simulink model "sampleModel62"  (R2021b)
settings: Solver=VariableStepAuto  StartTime=0.0  StopTime=10.0  RelTol=1e-3
undefined symbols (not defined in the file or in its folder): DiscIntNeverNeededParam, Newton, Raphson
libraries: simulink x13, slpidlib x3
settings Model: Creator=user  LastModifiedBy=user

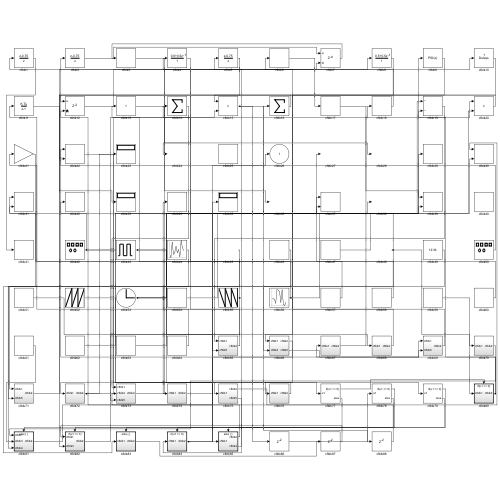
[thumbnail: Simulink's stored preview of the top-level diagram]
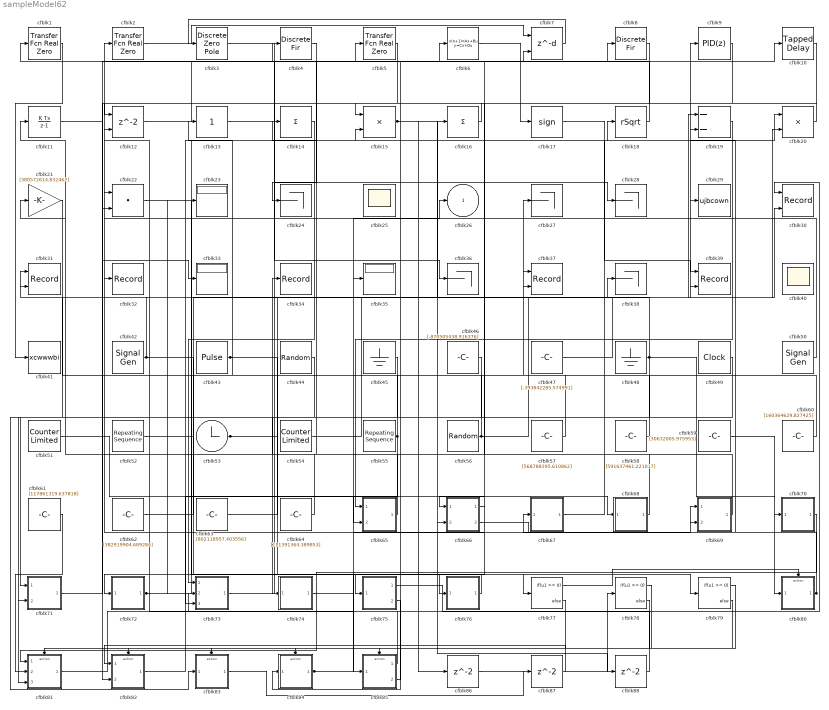
== system sampleModel62 ==
  cfblk1 : simulink/Discrete/Transfer Fcn Real Zero  ZeroZ=0.75  ICPrevInput=0.0  DoSatur=off
      settings: SourceProductBaseCode=SL
  cfblk10 : simulink/Discrete/Tapped Delay  vinit=0.0  samptime=-1  NumDelays=1  DelayOrder=Oldest  includeCurrent=off
  cfblk11 : DiscreteIntegrator  ICPrevOutput=DiscIntNeverNeededParam  ICPrevScaledInput=DiscIntNeverNeededParam
  cfblk12 : Delay  ShowEnablePort=on  SampleTime=1
      settings: InputPortMap=u0,e6
  cfblk13 : simulink/Math Operations/Slider Gain  gain=1  low=0  high=2
  cfblk14 : Sum  Inputs=+
  cfblk15 : Product  Inputs=**
  cfblk16 : Sum  Inputs=+
  cfblk17 : Signum
  cfblk18 : Sqrt  Operator=rSqrt  AlgorithmType=Newton-Raphson  SaturateOnIntegerOverflow=on
  cfblk19 : Sum  Inputs=--
  cfblk2 : simulink/Discrete/Transfer Fcn Real Zero  ZeroZ=0.75  ICPrevInput=0.0  DoSatur=off
      settings: SourceProductBaseCode=SL
  cfblk20 : Product
  cfblk21 : Gain  Gain=[380572614.832462]
  cfblk22 : DotProduct  InputSameDT=on  OutDataTypeStr=Inherit: Inherit via internal rule
  cfblk23 : Display
  cfblk{24,27..28,36,38} (5 alike) : Terminator
  cfblk25 : Scope
      settings: Floating=on
  cfblk29 : ToWorkspace  VariableName=ujbcown  SaveFormat=Timeseries  SampleTime=-1
  cfblk3 : DiscreteZeroPole  Poles=[0 0.5]  Gain=1
  cfblk30 : Record  FileSettingsInternal="{\"entries\":[{\"content\":{\"excelSettings\":{\"content\":{},\"type\":\"Streamout.ExcelSettings\"}},\"type\":\"Streamout.FileSettingStorage\",\"uuid\":\"89eb56b7-994b-4e5f-b351-745c7f58222d\"}],\"packageUris\":[\"http://schema.mathworks.com/mf0/streamout_blocks/R2020a\"],\"version\":\"1.0\"}"  Layout=[1 1]  SignalsInternal="{\"entries\":[{\"content\":{\"signals\":[{\"content\":{\"blockPath\":[\"sampleModel62/cfblk30\"],\"channel\":[],\"dimensions\":[1],\"domain\":\"sampleModel62/cfblk30\",\"lineColor\":\"#a2142f\",\"plots\":[1],\"port\":1,\"sid\":[\"\"],\"signalID\":2350,\"signalName\":\"cfblk75:1\"},\"type\":\"RecordBlkView.Signal\",\"uuid\":\"f3c1887c-4a82-4427-9ec1-d434c2a35077\"},{\"content\":{\"blockPath\":[\"sampleModel62/cfblk30\"],\"channel\":[],\"dimensions\":[1],\"domain\":\"sampleModel62/cfblk30\",\"lineColor\":\"#139fff\",\"plots\":[1],\"port\":2,\"sid\":[\"\"],\"signalID\":2354,\"signalName\":\"cfblk63\"},\"type\":\"RecordBlkView.Signal\",\"uuid\":\"385a4724-a655-411b-bda6-826876e1cbda\"}]},\"type\":\"RecordBlkView.InputSignals\",\"uuid\":\"7558fc44-3582-4613-9d91-3a130f029995\"}],\"packageUris\":[\"http://schema.mathworks.com/mf0/streamout_blocks/R2020a\"],\"version\":\"1.0\"}"  VisualizationBindings="{\"xyplotplugin\":{\"info\":[{\"series\":[{\"bindingParametersList\":[{\"parameter\":\"X-Axis\",\"signalID\":2350,\"signalName\":\"cfblk75:1\"},{\"parameter\":\"Y-Axis\",\"signalID\":2354,\"signalName\":\"cfblk63\"}],\"seriesID\":61633}],\"subplotID\":1}]}}"  CompatibilityTag=XY
  cfblk31 : Record  FileSettingsInternal="{\"entries\":[{\"content\":{\"excelSettings\":{\"content\":{},\"type\":\"Streamout.ExcelSettings\"}},\"type\":\"Streamout.FileSettingStorage\",\"uuid\":\"f6cec285-720d-4525-9b6c-a4037b512930\"}],\"packageUris\":[\"http://schema.mathworks.com/mf0/streamout_blocks/R2020a\"],\"version\":\"1.0\"}"  Layout=[1 1]  SignalsInternal="{\"entries\":[{\"content\":{\"signals\":[{\"content\":{\"blockPath\":[\"sampleModel62/cfblk31\"],\"channel\":[],\"dimensions\":[1],\"domain\":\"sampleModel62/cfblk31\",\"lineColor\":\"#139fff\",\"plots\":[1],\"port\":2,\"sid\":[\"\"],\"signalID\":2358,\"signalName\":\"cfblk55\"},\"type\":\"RecordBlkView.Signal\",\"uuid\":\"d1fee35e-af1c-4f30-8687-2a69d052420d\"},{\"content\":{\"blockPath\":[\"sampleModel62/cfblk31\"],\"channel\":[],\"dimensions\":[1],\"domain\":\"sampleModel62/cfblk31\",\"lineColor\":\"#a2142f\",\"plots\":[1],\"port\":1,\"sid\":[\"\"],\"signalID\":2387,\"signalName\":\"cfblk48\"},\"type\":\"RecordBlkView.Signal\",\"uuid\":\"631cae6d-1497-4714-8444-bf8a72d95f18\"}]},\"type\":\"RecordBlkView.InputSignals\",\"uuid\":\"f42cc6f8-42d1-4500-9fe3-c826577c401c\"}],\"packageUris\":[\"http://schema.mathworks.com/mf0/streamout_blocks/R2020a\"],\"version\":\"1.0\"}"  VisualizationBindings="{\"xyplotplugin\":{\"info\":[{\"series\":[{\"bindingParametersList\":[{\"parameter\":\"X-Axis\",\"signalID\":2387,\"signalName\":\"cfblk48\"},{\"parameter\":\"Y-Axis\",\"signalID\":2358,\"signalName\":\"cfblk55\"}],\"seriesID\":38390}],\"subplotID\":1}]}}"  CompatibilityTag=XY
  cfblk32 : Record  FileSettingsInternal="{\"entries\":[{\"content\":{\"excelSettings\":{\"content\":{},\"type\":\"Streamout.ExcelSettings\"}},\"type\":\"Streamout.FileSettingStorage\",\"uuid\":\"df777cac-f67f-4321-93c4-c3085ae9d89e\"}],\"packageUris\":[\"http://schema.mathworks.com/mf0/streamout_blocks/R2020a\"],\"version\":\"1.0\"}"  SignalsInternal="{\"entries\":[{\"content\":{\"signals\":[{\"content\":{\"blockPath\":[\"sampleModel62/cfblk32\"],\"channel\":[],\"dimensions\":[1],\"domain\":\"sampleModel62/cfblk32\",\"lineColor\":\"#4dbeee\",\"plots\":[1],\"port\":1,\"sid\":[\"\"],\"signalID\":2362,\"signalName\":\"cfblk42\"},\"type\":\"RecordBlkView.Signal\",\"uuid\":\"626f9505-6f8f-4dba-a9da-f5accb2c22b1\"}]},\"type\":\"RecordBlkView.InputSignals\",\"uuid\":\"e07a94e3-aac2-4026-a291-09599d10645f\"}],\"packageUris\":[\"http://schema.mathworks.com/mf0/streamout_blocks/R2020a\"],\"version\":\"1.0\"}"  VisualizationBindings="{\"sparklinesplugin\":{\"info\":[{\"bindingParametersList\":[],\"subplotID\":1}]}}"
  cfblk33 : Display
  cfblk34 : Record  FileSettingsInternal="{\"entries\":[{\"content\":{\"excelSettings\":{\"content\":{},\"type\":\"Streamout.ExcelSettings\"}},\"type\":\"Streamout.FileSettingStorage\",\"uuid\":\"2bc6c3f6-12ec-4b80-a0fb-0b9bce1de945\"}],\"packageUris\":[\"http://schema.mathworks.com/mf0/streamout_blocks/R2020a\"],\"version\":\"1.0\"}"  SignalsInternal="{\"entries\":[{\"content\":{\"signals\":[{\"content\":{\"blockPath\":[\"sampleModel62/cfblk34\"],\"channel\":[],\"dimensions\":[1],\"domain\":\"sampleModel62/cfblk34\",\"lineColor\":\"#64d413\",\"plots\":[1],\"port\":1,\"sid\":[\"\"],\"signalID\":2383,\"signalName\":\"cfblk64\"},\"type\":\"RecordBlkView.Signal\",\"uuid\":\"675a0413-753e-4dd3-8007-865c7edc0652\"}]},\"type\":\"RecordBlkView.InputSignals\",\"uuid\":\"41db974b-5a36-4903-a13c-916a7d049220\"}],\"packageUris\":[\"http://schema.mathworks.com/mf0/streamout_blocks/R2020a\"],\"version\":\"1.0\"}"  VisualizationBindings="{\"sparklinesplugin\":{\"info\":[{\"bindingParametersList\":[],\"subplotID\":1}]}}"
  cfblk35 : Display
  cfblk37 : Record  FileSettingsInternal="{\"entries\":[{\"content\":{\"excelSettings\":{\"content\":{},\"type\":\"Streamout.ExcelSettings\"}},\"type\":\"Streamout.FileSettingStorage\",\"uuid\":\"e84e0a09-953a-4701-9fb7-58381991c420\"}],\"packageUris\":[\"http://schema.mathworks.com/mf0/streamout_blocks/R2020a\"],\"version\":\"1.0\"}"  Layout=[1 1]  SignalsInternal="{\"entries\":[{\"content\":{\"signals\":[{\"content\":{\"blockPath\":[\"sampleModel62/cfblk37\"],\"channel\":[],\"dimensions\":[1],\"domain\":\"sampleModel62/cfblk37\",\"lineColor\":\"#a2142f\",\"plots\":[1],\"port\":1,\"sid\":[\"\"],\"signalID\":2366,\"signalName\":\"cfblk62\"},\"type\":\"RecordBlkView.Signal\",\"uuid\":\"9a5a44db-a54e-4c55-987a-8794391962ac\"},{\"content\":{\"blockPath\":[\"sampleModel62/cfblk37\"],\"channel\":[],\"dimensions\":[1],\"domain\":\"sampleModel62/cfblk37\",\"lineColor\":\"#139fff\",\"plots\":[1],\"port\":2,\"sid\":[\"\"],\"signalID\":2370,\"signalName\":\"cfblk53\"},\"type\":\"RecordBlkView.Signal\",\"uuid\":\"b6f7ba66-1672-4726-bd48-e830112b5529\"}]},\"type\":\"RecordBlkView.InputSignals\",\"uuid\":\"db1642b9-4836-40d2-9913-e3669089fdb1\"}],\"packageUris\":[\"http://schema.mathworks.com/mf0/streamout_blocks/R2020a\"],\"version\":\"1.0\"}"  VisualizationBindings="{\"xyplotplugin\":{\"info\":[{\"series\":[{\"bindingParametersList\":[{\"parameter\":\"X-Axis\",\"signalID\":2366,\"signalName\":\"cfblk62\"},{\"parameter\":\"Y-Axis\",\"signalID\":2370,\"signalName\":\"cfblk53\"}],\"seriesID\":30424}],\"subplotID\":1}]}}"  CompatibilityTag=XY
  cfblk39 : Record  FileSettingsInternal="{\"entries\":[{\"content\":{\"excelSettings\":{\"content\":{},\"type\":\"Streamout.ExcelSettings\"}},\"type\":\"Streamout.FileSettingStorage\",\"uuid\":\"19a212e9-ba54-497d-8557-3380ead62d9a\"}],\"packageUris\":[\"http://schema.mathworks.com/mf0/streamout_blocks/R2020a\"],\"version\":\"1.0\"}"  Layout=[1 1]  SignalsInternal="{\"entries\":[{\"content\":{\"signals\":[{\"content\":{\"blockPath\":[\"sampleModel62/cfblk39\"],\"channel\":[],\"dimensions\":[1],\"domain\":\"sampleModel62/cfblk39\",\"lineColor\":\"#a2142f\",\"plots\":[1],\"port\":1,\"sid\":[\"\"],\"signalID\":2374,\"signalName\":\"cfblk17\"},\"type\":\"RecordBlkView.Signal\",\"uuid\":\"715f0c9c-babd-4185-9a5d-3f6c9038a850\"},{\"content\":{\"blockPath\":[\"sampleModel62/cfblk39\"],\"channel\":[],\"dimensions\":[1],\"domain\":\"sampleModel62/cfblk39\",\"lineColor\":\"#139fff\",\"plots\":[1],\"port\":2,\"sid\":[\"\"],\"signalID\":2379,\"signalName\":\"cfblk54\"},\"type\":\"RecordBlkView.Signal\",\"uuid\":\"af095b9f-c74a-41a2-9f00-3ee94e8c8fd4\"}]},\"type\":\"RecordBlkView.InputSignals\",\"uuid\":\"4e895160-30f6-4ff3-8ca9-daca12cead85\"}],\"packageUris\":[\"http://schema.mathworks.com/mf0/streamout_blocks/R2020a\"],\"version\":\"1.0\"}"  VisualizationBindings="{\"xyplotplugin\":{\"info\":[{\"series\":[{\"bindingParametersList\":[{\"parameter\":\"X-Axis\",\"signalID\":2374,\"signalName\":\"cfblk17\"},{\"parameter\":\"Y-Axis\",\"signalID\":2379,\"signalName\":\"cfblk54\"}],\"seriesID\":1351}],\"subplotID\":1}]}}"  CompatibilityTag=XY
  cfblk4 : DiscreteFir  SampleTime=1
  cfblk40 : Scope
      settings: Floating=on
  cfblk41 : ToWorkspace  VariableName=xcwwwbi  SaveFormat=Timeseries  SampleTime=-1
  cfblk42 : SignalGenerator  WaveForm=sawtooth  Amplitude=[-543573503.028565]  Units=rad/sec
  cfblk43 : DiscretePulseGenerator  PulseType=Time based  Amplitude=[762596451.734230]  Period=[19367313.235123]  PulseWidth=5  PhaseDelay=[8.000000]
  cfblk44 : UniformRandomNumber  Minimum=[-7920190339.645073]  Maximum=[6705395150.499472]  Seed=[21644592.000000]  SampleTime=0.1
  cfblk45 : Ground
  cfblk46 : Constant  Value=[-870505438.916376]  SampleTime=1
  cfblk47 : Constant  Value=[-393842285.574991]  SampleTime=1
  cfblk48 : Ground
  cfblk49 : DigitalClock
  cfblk5 : simulink/Discrete/Transfer Fcn Real Zero  ZeroZ=0.75  ICPrevInput=0.0  DoSatur=off
      settings: SourceProductBaseCode=SL
  cfblk50 : SignalGenerator  WaveForm=sawtooth  Amplitude=[-508428864.586431]  Units=rad/sec
  cfblk51 : simulink/Sources/Counter Limited  uplimit=[1.000000]  tsamp=-1
  cfblk52 : simulink/Sources/Repeating Sequence  rep_seq_t=[0 2]  rep_seq_y=[-994144849.928025, 851397030.625694]
  cfblk53 : Clock
  cfblk54 : simulink/Sources/Counter Limited  uplimit=[40.000000]  tsamp=-1
  cfblk55 : simulink/Sources/Repeating Sequence  rep_seq_t=[0 2]  rep_seq_y=[74149464.534374, -616770878.881431]
  cfblk56 : RandomNumber  Mean=[-67269.871624]  Variance=[69724.484070]  Seed=[668721954.000000]  SampleTime=0.1
  cfblk57 : Constant  Value=[568788395.610862]  SampleTime=1
  cfblk58 : Constant  Value=[591637461.221017]  SampleTime=1
  cfblk59 : Constant  Value=[30632005.975953]  SampleTime=1
  cfblk6 : DiscreteStateSpace
  cfblk60 : Constant  Value=[160364629.827425]  SampleTime=1
  cfblk61 : Constant  Value=[117861319.637818]  SampleTime=1
  cfblk62 : Constant  Value=[382919904.689284]  SampleTime=1
  cfblk63 : Constant  Value=[802118957.403556]  SampleTime=1
  cfblk64 : Constant  Value=[111391364.389853]  SampleTime=1
  cfblk65 : Subsystem
  cfblk66 : Subsystem
  cfblk67 : Subsystem
  cfblk68 : Subsystem
  cfblk69 : Subsystem
  cfblk7 : Delay  DelayLengthSource=Input port  SampleTime=1
      settings: InputPortMap=u0,p1
  cfblk70 : Subsystem
  cfblk71 : Subsystem
  cfblk72 : Subsystem
  cfblk73 : Subsystem
  cfblk74 : Subsystem
  cfblk75 : Subsystem
  cfblk76 : Subsystem
  cfblk77 : If  IfExpression=u1 >= 0  SampleTime=1
  cfblk78 : If  IfExpression=u1 >= 0  SampleTime=1
  cfblk79 : If  IfExpression=u1 >= 0  SampleTime=1
  cfblk8 : DiscreteFir  SampleTime=1
  cfblk80 : Subsystem  TreatAsAtomicUnit=on
  cfblk81 : Subsystem  TreatAsAtomicUnit=on
  cfblk82 : Subsystem  TreatAsAtomicUnit=on
  cfblk83 : Subsystem  TreatAsAtomicUnit=on
  cfblk84 : Subsystem  TreatAsAtomicUnit=on
  cfblk85 : Subsystem  TreatAsAtomicUnit=on
  cfblk86 : Delay  SampleTime=1
  cfblk87 : Delay  SampleTime=1
  cfblk88 : Delay  SampleTime=1
  cfblk9 : slpidlib/PID Controller  Controller=PID  Form=Parallel  TimeDomain=Discrete-time  UseExternalTs=off  SampleTime=1  IntegratorMethod=Forward Euler  FilterMethod=Forward Euler  ControllerParametersSource=internal  P=1  I=1  D=0  UseFilter=on  N=100  TunerSelectOption=Transfer Function Based (PID Tuner App)  InitialConditionSource=internal  InitialConditionForIntegrator=0  InitialConditionForFilter=0  DifferentiatorICPrevScaledInput=0  ExternalReset=none  TrackingMode=off  Kt=1  LimitOutput=off  SatLimitsSource=internal  UpperSaturationLimit=inf  LowerSaturationLimit=-inf  LinearizeAsGain=off  AntiWindupMode=none  Kb=1  POutMin=[]  POutMax=[]  IOutMin=[]  IOutMax=[]  DOutMin=[]  DOutMax=[]  NOutMin=[]  NOutMax=[]  SumOutMin=[]  SumOutMax=[]  SaturationOutMin=[]  SaturationOutMax=[]  PParamMin=[]  PParamMax=[]  IParamMin=[]  IParamMax=[]  DParamMin=[]  DParamMax=[]  NParamMin=[]  NParamMax=[]  KbParamMin=[]  KbParamMax=[]  KtParamMin=[]  KtParamMax=[]  KbOutMin=[]  KbOutMax=[]  KtOutMin=[]  KtOutMax=[]  IntegratorOutMin=[]  IntegratorOutMax=[]  FilterOutMin=[]  FilterOutMax=[]  SumI1OutMin=[]  SumI1OutMax=[]  SumI2OutMin=[]  SumI2OutMax=[]  SumI3OutMin=[]  SumI3OutMax=[]  SumI4OutMin=[]  SumI4OutMax=[]  SumDOutMin=[]  SumDOutMax=[]  DifferentiatorOutMin=[]  DifferentiatorOutMax=[]  FilterDiffOutCoefMin=[]  FilterDiffOutCoefMax=[]  ReciprocalOutMin=[]  ReciprocalOutMax=[]  SumDenOutMin=[]  SumDenOutMax=[]  SumNumOutMin=[]  SumNumOutMax=[]  DivideOutMin=[]  DivideOutMax=[]  UdiffTsProdOutMin=[]  UdiffTsProdOutMax=[]  NTsProdOutMin=[]  NTsProdOutMax=[]  UintegralTsProdOutMin=[]  UintegralTsProdOutMax=[]  UngainTsProdOutMin=[]  UngainTsProdOutMax=[]  IntegratorContinuousStateAttributes=''  IntegratorStateMustResolveToSignalObject=off  IntegratorRTWStateStorageClass=Auto  FilterContinuousStateAttributes=''  FilterStateMustResolveToSignalObject=off  FilterRTWStateStorageClass=Auto  ParallelPVariant=InternalParameters  IdealPVariant=Disabled  IVariant=InternalParameters  DVariant=InternalParameters  IntegratorVariant=Discrete  SatVariant=Disabled  AWVariant=Passthrough  PCopyVariant=Disabled  TRVariant=Disabled  FdbkBlocksVariant=Forward  IdealPFdbkVariant=Disabled  SatFdbkVariant=Disabled  DerivativeFilterVariant=ForwardEulerFilter  NVariant=InternalParameters  NCopyVariant=Disabled  FilterICVariant=InternalICsFilter  IntegratorICVariant=InternalICs  ExternalResetVariant=Disabled  TRSumVariant=Passthrough  SumFdbkVariant=Disabled  SumVariant=Sum_PID  TsampFilterVariant=InternalTs  TsampNgainVariant=Passthrough  TsampIntegralVariant=Passthrough  ExternalSaturationOutDataTypeStr=Inherit: Same as second input
  cfblk26 : Outport
  wires:
  cfblk19/1 -> cfblk65/1(cfblk1)
  cfblk2/1 -> cfblk7/1
  cfblk42/1 -> cfblk9/1, cfblk32/1, cfblk77/1
  cfblk66/1(cfblk2) -> cfblk2/1
  cfblk47/1 -> cfblk29/1
  cfblk73/1(cfblk2) -> cfblk7/2
  cfblk70/1(cfblk2) -> cfblk81/1(cfblk1)
  cfblk12/1 -> cfblk10/1
  cfblk44/1 -> cfblk74/1(cfblk1)
  cfblk59/1 -> cfblk80/1(cfblk1)
  cfblk72/1(cfblk2) -> cfblk18/1, cfblk23/1
  cfblk13/1 -> cfblk36/1
  cfblk15/1 -> cfblk86/1, cfblk88/1
  cfblk17/1 -> cfblk39/1
  cfblk61/1 -> cfblk81/2(cfblk3)
  cfblk16/1 -> cfblk12/1
  cfblk76/1(cfblk2) -> cfblk72/1(cfblk1)
  cfblk81/1(cfblk2) -> cfblk35/1
  cfblk21/1 -> cfblk83/1(cfblk1)
  cfblk48/1 -> cfblk31/1, cfblk71/2(cfblk5), cfblk70/1(cfblk1)
  cfblk43/1 -> cfblk68/1(cfblk1), cfblk79/1
  cfblk68/1(cfblk2) -> cfblk21/1
  cfblk45/1 -> cfblk71/1(cfblk1)
  cfblk50/1 -> cfblk22/1
  cfblk64/1 -> cfblk34/1
  cfblk52/1 -> cfblk75/1(cfblk1)
  cfblk85/1(cfblk2) -> cfblk12/2
  cfblk53/1 -> cfblk16/1, cfblk37/2, cfblk19/1
  cfblk7/1 -> cfblk3/1
  cfblk69/1(cfblk2) -> cfblk6/1
  cfblk20/1 -> cfblk15/1
  cfblk5/1 -> cfblk22/2
  cfblk10/1 -> cfblk82/2(cfblk3)
  cfblk3/1 -> cfblk28/1
  cfblk8/1 -> cfblk66/1(cfblk1)
  cfblk75/1(cfblk2) -> cfblk30/1
  cfblk71/1(cfblk2) -> cfblk8/1
  cfblk63/1 -> cfblk30/2
  cfblk1/1 -> cfblk41/1
  cfblk54/1 -> cfblk39/2
  cfblk65/1(cfblk2) -> cfblk4/1
  cfblk14/1 -> cfblk73/1(cfblk1)
  cfblk49/1 -> cfblk81/3(cfblk4)
  cfblk67/1(cfblk2) -> cfblk20/1
  cfblk75/2(cfblk5) -> cfblk84/1(cfblk1)
  cfblk55/1 -> cfblk31/2, cfblk73/3(cfblk5)
  cfblk22/1 -> cfblk85/1(cfblk1)
  cfblk56/1 -> cfblk20/2, cfblk11/1
  cfblk58/1 -> cfblk27/1
  cfblk57/1 -> cfblk14/1
  cfblk9/1 -> cfblk76/1(cfblk1)
  cfblk18/1 -> cfblk1/1
  cfblk62/1 -> cfblk37/1
  cfblk74/1(cfblk2) -> cfblk69/1(cfblk1)
  cfblk80/1(cfblk2) -> cfblk67/1(cfblk1), cfblk19/2
  cfblk11/1 -> cfblk33/1
  cfblk60/1 -> cfblk13/1
  cfblk84/1(cfblk2) -> cfblk38/1, cfblk26/1
  cfblk66/2(cfblk5) -> cfblk69/2(cfblk5)
  cfblk6/1 -> cfblk17/1
  cfblk82/1(cfblk2) -> cfblk15/2
  cfblk51/1 -> cfblk65/2(cfblk5)
  cfblk4/1 -> cfblk24/1
  cfblk46/1 -> cfblk66/2(cfblk4)
  cfblk85/2(cfblk4) -> cfblk73/2(cfblk4)
  cfblk77/1 -> cfblk80/Action
  cfblk77/2 -> cfblk81/Action
  cfblk78/1 -> cfblk82/Action
  cfblk78/2 -> cfblk83/Action
  cfblk79/1 -> cfblk84/Action
  cfblk79/2 -> cfblk85/Action
  cfblk86/1 -> cfblk78/1
  cfblk83/1(cfblk2) -> cfblk87/1
  cfblk87/1 -> cfblk82/1(cfblk1)
  cfblk88/1 -> cfblk5/1

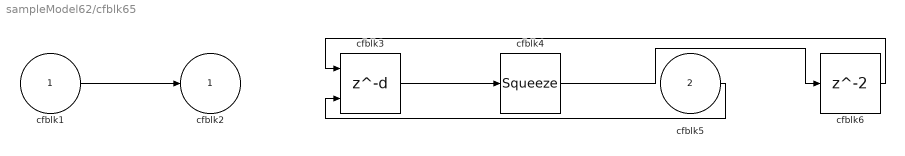
== system sampleModel62/cfblk65 ==
  cfblk1 : Inport
  cfblk5 : Inport  Port=2
  cfblk3 : Delay  DelayLengthSource=Input port  SampleTime=1
      settings: InputPortMap=u0,p1
  cfblk4 : Squeeze
  cfblk6 : Delay  SampleTime=1
  cfblk2 : Outport
  wires:
  cfblk5/1 -> cfblk3/2
  cfblk3/1 -> cfblk4/1
  cfblk1/1 -> cfblk2/1
  cfblk4/1 -> cfblk6/1
  cfblk6/1 -> cfblk3/1

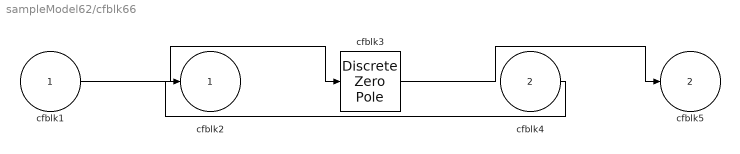
== system sampleModel62/cfblk66 ==
  cfblk1 : Inport
  cfblk4 : Inport  Port=2
  cfblk3 : DiscreteZeroPole  Poles=[0 0.5]  Gain=1
  cfblk2 : Outport
  cfblk5 : Outport  Port=2
  wires:
  cfblk1/1 -> cfblk3/1
  cfblk3/1 -> cfblk5/1
  cfblk4/1 -> cfblk2/1

== system sampleModel62/cfblk67 ==
  cfblk1 : Inport
  cfblk3 : DiscreteIntegrator  ICPrevOutput=DiscIntNeverNeededParam  ICPrevScaledInput=DiscIntNeverNeededParam
  cfblk4 : slpidlib/PID Controller  Controller=PID  Form=Parallel  TimeDomain=Discrete-time  UseExternalTs=off  SampleTime=1  IntegratorMethod=Forward Euler  FilterMethod=Forward Euler  ControllerParametersSource=internal  P=1  I=1  D=0  UseFilter=on  N=100  TunerSelectOption=Transfer Function Based (PID Tuner App)  InitialConditionSource=internal  InitialConditionForIntegrator=0  InitialConditionForFilter=0  DifferentiatorICPrevScaledInput=0  ExternalReset=none  TrackingMode=off  Kt=1  LimitOutput=off  SatLimitsSource=internal  UpperSaturationLimit=inf  LowerSaturationLimit=-inf  LinearizeAsGain=off  AntiWindupMode=none  Kb=1  POutMin=[]  POutMax=[]  IOutMin=[]  IOutMax=[]  DOutMin=[]  DOutMax=[]  NOutMin=[]  NOutMax=[]  SumOutMin=[]  SumOutMax=[]  SaturationOutMin=[]  SaturationOutMax=[]  PParamMin=[]  PParamMax=[]  IParamMin=[]  IParamMax=[]  DParamMin=[]  DParamMax=[]  NParamMin=[]  NParamMax=[]  KbParamMin=[]  KbParamMax=[]  KtParamMin=[]  KtParamMax=[]  KbOutMin=[]  KbOutMax=[]  KtOutMin=[]  KtOutMax=[]  IntegratorOutMin=[]  IntegratorOutMax=[]  FilterOutMin=[]  FilterOutMax=[]  SumI1OutMin=[]  SumI1OutMax=[]  SumI2OutMin=[]  SumI2OutMax=[]  SumI3OutMin=[]  SumI3OutMax=[]  SumI4OutMin=[]  SumI4OutMax=[]  SumDOutMin=[]  SumDOutMax=[]  DifferentiatorOutMin=[]  DifferentiatorOutMax=[]  FilterDiffOutCoefMin=[]  FilterDiffOutCoefMax=[]  ReciprocalOutMin=[]  ReciprocalOutMax=[]  SumDenOutMin=[]  SumDenOutMax=[]  SumNumOutMin=[]  SumNumOutMax=[]  DivideOutMin=[]  DivideOutMax=[]  UdiffTsProdOutMin=[]  UdiffTsProdOutMax=[]  NTsProdOutMin=[]  NTsProdOutMax=[]  UintegralTsProdOutMin=[]  UintegralTsProdOutMax=[]  UngainTsProdOutMin=[]  UngainTsProdOutMax=[]  IntegratorContinuousStateAttributes=''  IntegratorStateMustResolveToSignalObject=off  IntegratorRTWStateStorageClass=Auto  FilterContinuousStateAttributes=''  FilterStateMustResolveToSignalObject=off  FilterRTWStateStorageClass=Auto  ParallelPVariant=InternalParameters  IdealPVariant=Disabled  IVariant=InternalParameters  DVariant=InternalParameters  IntegratorVariant=Discrete  SatVariant=Disabled  AWVariant=Passthrough  PCopyVariant=Disabled  TRVariant=Disabled  FdbkBlocksVariant=Forward  IdealPFdbkVariant=Disabled  SatFdbkVariant=Disabled  DerivativeFilterVariant=ForwardEulerFilter  NVariant=InternalParameters  NCopyVariant=Disabled  FilterICVariant=InternalICsFilter  IntegratorICVariant=InternalICs  ExternalResetVariant=Disabled  TRSumVariant=Passthrough  SumFdbkVariant=Disabled  SumVariant=Sum_PID  TsampFilterVariant=InternalTs  TsampNgainVariant=Passthrough  TsampIntegralVariant=Passthrough  ExternalSaturationOutDataTypeStr=Inherit: Same as second input
  cfblk2 : Outport
  wires:
  cfblk1/1 -> cfblk4/1
  cfblk3/1 -> cfblk2/1
  cfblk4/1 -> cfblk3/1

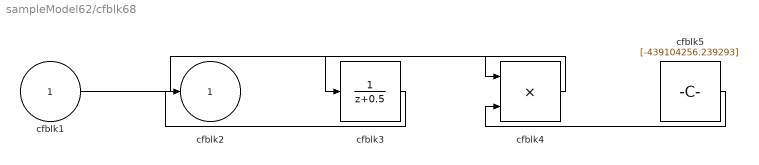
== system sampleModel62/cfblk68 ==
  cfblk1 : Inport
  cfblk3 : DiscreteTransferFcn  SampleTime=1
  cfblk4 : Product  Inputs=**
  cfblk5 : Constant  Value=[-439104256.239293]  SampleTime=1
  cfblk2 : Outport
  wires:
  cfblk1/1 -> cfblk4/1
  cfblk5/1 -> cfblk4/2
  cfblk4/1 -> cfblk3/1
  cfblk3/1 -> cfblk2/1

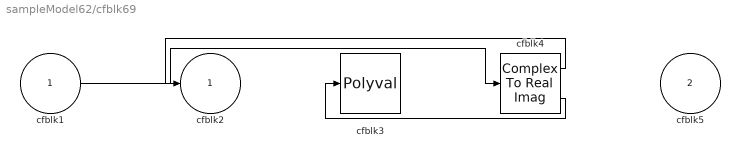
== system sampleModel62/cfblk69 ==
  cfblk1 : Inport
  cfblk5 : Inport  Port=2
  cfblk3 : Polyval  Coefs=[ +2.081618890e-019, -1.441693666e-014, +4.719686976e-010, -8.536869453e-006, +1.621573104e-001, -8.087801117e+001 ]
  cfblk4 : ComplexToRealImag
  cfblk2 : Outport
  wires:
  cfblk1/1 -> cfblk4/1
  cfblk4/1 -> cfblk2/1
  cfblk4/2 -> cfblk3/1

== system sampleModel62/cfblk70 ==
  cfblk1 : Inport
  cfblk3 : simulink/Math Operations/MinMax Running Resettable  Function=min  vinit=0.0
  cfblk4 : Polyval  Coefs=[ +2.081618890e-019, -1.441693666e-014, +4.719686976e-010, -8.536869453e-006, +1.621573104e-001, -8.087801117e+001 ]
  cfblk2 : Outport
  wires:
  cfblk4/1 -> cfblk3/1, cfblk3/2
  cfblk1/1 -> cfblk4/1
  cfblk3/1 -> cfblk2/1

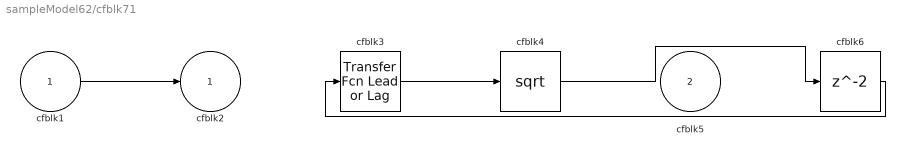
== system sampleModel62/cfblk71 ==
  cfblk1 : Inport
  cfblk5 : Inport  Port=2
  cfblk3 : simulink/Discrete/Transfer Fcn Lead or Lag  PoleZ=0.95  ZeroZ=0.75  ICPrevOutput=0.0  ICPrevInput=0.0  DoSatur=off
      settings: SourceProductBaseCode=SL
  cfblk4 : Sqrt  SaturateOnIntegerOverflow=on
  cfblk6 : Delay  SampleTime=1
  cfblk2 : Outport
  wires:
  cfblk3/1 -> cfblk4/1
  cfblk1/1 -> cfblk2/1
  cfblk4/1 -> cfblk6/1
  cfblk6/1 -> cfblk3/1

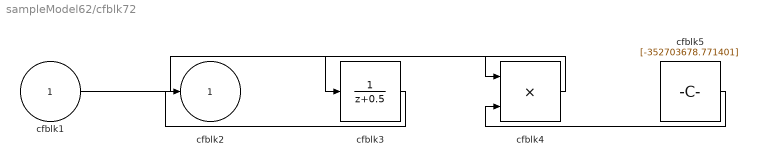
== system sampleModel62/cfblk72 ==
  cfblk1 : Inport
  cfblk3 : DiscreteTransferFcn  SampleTime=1
  cfblk4 : Product
  cfblk5 : Constant  Value=[-352703678.771401]  SampleTime=1
  cfblk2 : Outport
  wires:
  cfblk1/1 -> cfblk4/1
  cfblk5/1 -> cfblk4/2
  cfblk4/1 -> cfblk3/1
  cfblk3/1 -> cfblk2/1

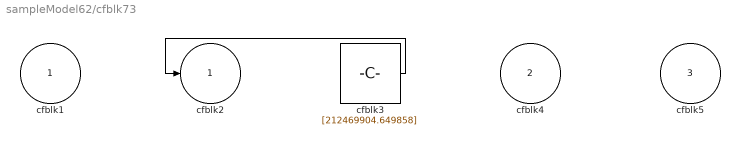
== system sampleModel62/cfblk73 ==
  cfblk1 : Inport
  cfblk4 : Inport  Port=2
  cfblk5 : Inport  Port=3
  cfblk3 : Constant  Value=[212469904.649858]  SampleTime=1
  cfblk2 : Outport
  wires:
  cfblk3/1 -> cfblk2/1

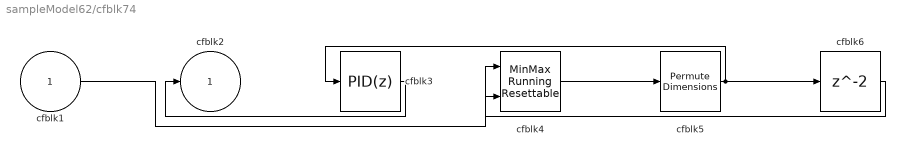
== system sampleModel62/cfblk74 ==
  cfblk1 : Inport
  cfblk3 : slpidlib/PID Controller  Controller=PID  Form=Parallel  TimeDomain=Discrete-time  UseExternalTs=off  SampleTime=1  IntegratorMethod=Forward Euler  FilterMethod=Forward Euler  ControllerParametersSource=internal  P=1  I=1  D=0  UseFilter=on  N=100  TunerSelectOption=Transfer Function Based (PID Tuner App)  InitialConditionSource=internal  InitialConditionForIntegrator=0  InitialConditionForFilter=0  DifferentiatorICPrevScaledInput=0  ExternalReset=none  TrackingMode=off  Kt=1  LimitOutput=off  SatLimitsSource=internal  UpperSaturationLimit=inf  LowerSaturationLimit=-inf  LinearizeAsGain=off  AntiWindupMode=none  Kb=1  POutMin=[]  POutMax=[]  IOutMin=[]  IOutMax=[]  DOutMin=[]  DOutMax=[]  NOutMin=[]  NOutMax=[]  SumOutMin=[]  SumOutMax=[]  SaturationOutMin=[]  SaturationOutMax=[]  PParamMin=[]  PParamMax=[]  IParamMin=[]  IParamMax=[]  DParamMin=[]  DParamMax=[]  NParamMin=[]  NParamMax=[]  KbParamMin=[]  KbParamMax=[]  KtParamMin=[]  KtParamMax=[]  KbOutMin=[]  KbOutMax=[]  KtOutMin=[]  KtOutMax=[]  IntegratorOutMin=[]  IntegratorOutMax=[]  FilterOutMin=[]  FilterOutMax=[]  SumI1OutMin=[]  SumI1OutMax=[]  SumI2OutMin=[]  SumI2OutMax=[]  SumI3OutMin=[]  SumI3OutMax=[]  SumI4OutMin=[]  SumI4OutMax=[]  SumDOutMin=[]  SumDOutMax=[]  DifferentiatorOutMin=[]  DifferentiatorOutMax=[]  FilterDiffOutCoefMin=[]  FilterDiffOutCoefMax=[]  ReciprocalOutMin=[]  ReciprocalOutMax=[]  SumDenOutMin=[]  SumDenOutMax=[]  SumNumOutMin=[]  SumNumOutMax=[]  DivideOutMin=[]  DivideOutMax=[]  UdiffTsProdOutMin=[]  UdiffTsProdOutMax=[]  NTsProdOutMin=[]  NTsProdOutMax=[]  UintegralTsProdOutMin=[]  UintegralTsProdOutMax=[]  UngainTsProdOutMin=[]  UngainTsProdOutMax=[]  IntegratorContinuousStateAttributes=''  IntegratorStateMustResolveToSignalObject=off  IntegratorRTWStateStorageClass=Auto  FilterContinuousStateAttributes=''  FilterStateMustResolveToSignalObject=off  FilterRTWStateStorageClass=Auto  ParallelPVariant=InternalParameters  IdealPVariant=Disabled  IVariant=InternalParameters  DVariant=InternalParameters  IntegratorVariant=Discrete  SatVariant=Disabled  AWVariant=Passthrough  PCopyVariant=Disabled  TRVariant=Disabled  FdbkBlocksVariant=Forward  IdealPFdbkVariant=Disabled  SatFdbkVariant=Disabled  DerivativeFilterVariant=ForwardEulerFilter  NVariant=InternalParameters  NCopyVariant=Disabled  FilterICVariant=InternalICsFilter  IntegratorICVariant=InternalICs  ExternalResetVariant=Disabled  TRSumVariant=Passthrough  SumFdbkVariant=Disabled  SumVariant=Sum_PID  TsampFilterVariant=InternalTs  TsampNgainVariant=Passthrough  TsampIntegralVariant=Passthrough  ExternalSaturationOutDataTypeStr=Inherit: Same as second input
  cfblk4 : simulink/Math Operations/MinMax Running Resettable  Function=min  vinit=0.0
  cfblk5 : PermuteDimensions
  cfblk6 : Delay  SampleTime=1
  cfblk2 : Outport
  wires:
  cfblk5/1 -> cfblk3/1, cfblk6/1
  cfblk3/1 -> cfblk2/1
  cfblk4/1 -> cfblk5/1
  cfblk1/1 -> cfblk4/1
  cfblk6/1 -> cfblk4/2

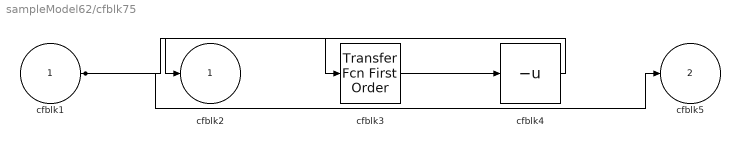
== system sampleModel62/cfblk75 ==
  cfblk1 : Inport
  cfblk3 : simulink/Discrete/Transfer Fcn First Order  PoleZ=0.95  ICPrevOutput=0.0  DoSatur=off
  cfblk4 : UnaryMinus
  cfblk2 : Outport
  cfblk5 : Outport  Port=2
  wires:
  cfblk4/1 -> cfblk2/1
  cfblk1/1 -> cfblk5/1, cfblk3/1
  cfblk3/1 -> cfblk4/1

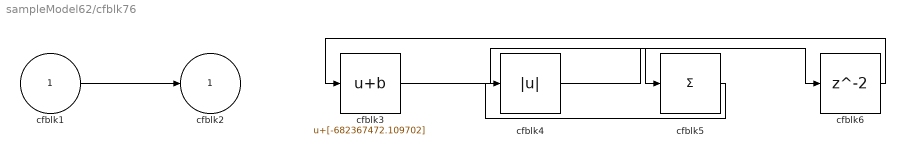
== system sampleModel62/cfblk76 ==
  cfblk1 : Inport
  cfblk3 : Bias  Bias=[-682367472.109702]
  cfblk4 : Abs
  cfblk5 : Sum  Inputs=+
  cfblk6 : Delay  SampleTime=1
  cfblk2 : Outport
  wires:
  cfblk3/1 -> cfblk5/1
  cfblk1/1 -> cfblk2/1
  cfblk5/1 -> cfblk4/1
  cfblk4/1 -> cfblk6/1
  cfblk6/1 -> cfblk3/1

== system sampleModel62/cfblk80 ==
  cfblk1 : Inport
  Action Port : ActionPort  ActionPortLabel=if(u1 >= 0)
  cfblk3 : Rounding
  cfblk2 : Outport
  wires:
  cfblk3/1 -> cfblk2/1
  cfblk1/1 -> cfblk3/1

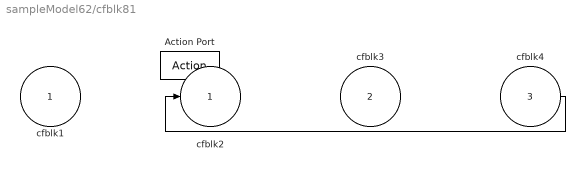
== system sampleModel62/cfblk81 ==
  cfblk1 : Inport
  cfblk3 : Inport  Port=2
  cfblk4 : Inport  Port=3
  Action Port : ActionPort  ActionPortLabel=else
  cfblk2 : Outport
  wires:
  cfblk4/1 -> cfblk2/1

== system sampleModel62/cfblk82 ==
  cfblk1 : Inport
  cfblk3 : Inport  Port=2
  Action Port : ActionPort  ActionPortLabel=if(u1 >= 0)
  cfblk2 : Outport
  wires:
  cfblk3/1 -> cfblk2/1

== system sampleModel62/cfblk83 ==
  cfblk1 : Inport
  Action Port : ActionPort  ActionPortLabel=else
  cfblk3 : UnitDelay  SampleTime=-1  HasFrameUpgradeWarning=on
  cfblk4 : Constant  Value=[-544751748.578219]  SampleTime=1
  cfblk2 : Outport
  wires:
  cfblk4/1 -> cfblk2/1
  cfblk1/1 -> cfblk3/1

== system sampleModel62/cfblk84 ==
  cfblk1 : Inport
  Action Port : ActionPort  ActionPortLabel=if(u1 >= 0)
  cfblk3 : Sum  Inputs=+-
  cfblk2 : Outport
  wires:
  cfblk1/1 -> cfblk3/1, cfblk3/2
  cfblk3/1 -> cfblk2/1

== system sampleModel62/cfblk85 ==
  cfblk1 : Inport
  Action Port : ActionPort  ActionPortLabel=else
  cfblk3 : DiscreteStateSpace  SampleTime=-1
  cfblk2 : Outport
  cfblk4 : Outport  Port=2
  wires:
  cfblk3/1 -> cfblk4/1, cfblk2/1
  cfblk1/1 -> cfblk3/1
